simulink model "Derivative_loop"  (R2020b)
settings: Solver=VariableStepAuto  StartTime=0.0  StopTime=10.0  RelTol=1e-3
values from neighbouring files (symbols this model uses):
  A = 2    [Control.m]
  F = 5    [Control.m]
  Ti = 4    [Control.m]
settings Model: Creator=Raihan mahmud  LastModifiedBy=Raihan mahmud

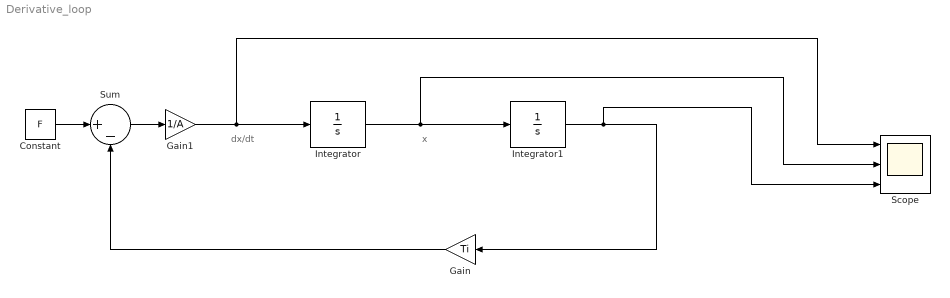
== system Derivative_loop ==
  note: x
  note: dx/dt
  Constant : Constant  Value=F
  Gain : Gain  Gain=Ti
  Gain1 : Gain  Gain=1/A
  Integrator : Integrator
  Integrator1 : Integrator
  Scope : Scope  NumInputPorts=3
  Sum : Sum  Inputs=|+-
  wires:
  Integrator1/1 -> Scope/3, Gain/1
  Constant/1 -> Sum/1
  Gain/1 -> Sum/2
  Sum/1 -> Gain1/1
  Integrator/1 -> Scope/2, Integrator1/1
  Gain1/1 -> Scope/1, Integrator/1
